simulink model "simscape_Example_20240513_1634"  (R2023b)
settings: Solver=ode23t  StartTime=0.0  StopTime=100  RelTol=1e-3
libraries: nesl_utility x10, fl_lib x8, ee_lib x4
settings Model: Creator=Patri  LastModifiedBy=Patri

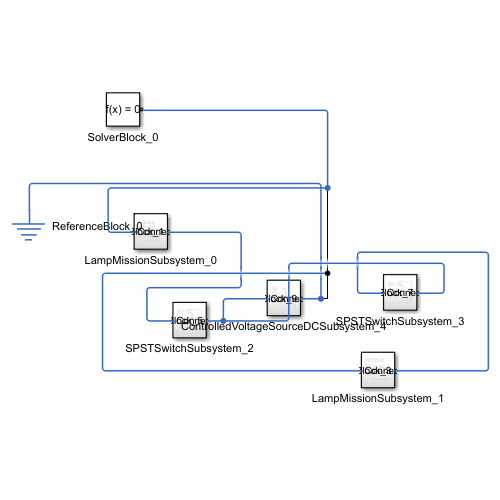
[thumbnail: Simulink's stored preview of the top-level diagram]
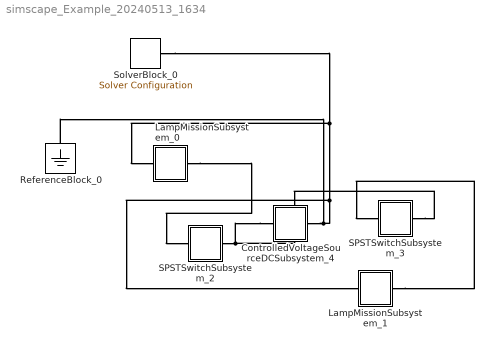
== system simscape_Example_20240513_1634 ==
  ControlledVoltageSourceDCSubsystem_4 : Subsystem
  LampMissionSubsystem_0 : Subsystem
  LampMissionSubsystem_1 : Subsystem
  ReferenceBlock_0 : fl_lib/Electrical/Electrical Elements/Electrical Reference
  SPSTSwitchSubsystem_2 : Subsystem
  SPSTSwitchSubsystem_3 : Subsystem
  SolverBlock_0 : nesl_utility/Solver Configuration  PhysicalDomain=network_engine_domain  SubClassName=solver  LeftPortType=input  RightPortType=generic  Tones=[]  Harmonics=[]  SimulateNoise=off  Profile=off  UseLocalSampling=off  EnableSwitchedLinearOptims=on  FrequencyDomain=off  UseCCode=off  RelTol=0.001  AbsTol=0.001  MinStep=1e-09  ToWorkspace=off  RevertToSquareIcSolve=off  NumHomotopyIterations=100  PhasorMode=off  PhasorModeNumHarmonics=1  ConsistencySolver=NEWTON_XTOL_AFTER_FTOL  IndexReductionMethod=DerivativeReplacement  DoDC=off  ResidualTolerance=1e-09  ConsistencyTolSource=GLOBAL  ConsistencyAbsTol=0.001  ConsistencyRelTol=0.001  ConsistencyTolFactor=0.001  UseLocalSolver=off  LocalSolverChoice=NE_BACKWARD_EULER_ADVANCER  ResolveIndetEquations=on  FunctionEvalNumThread=1  LocalSolverSampleTime=0.001  DoFixedCost=off  MaxNonlinIter=3  MaxModeIter=2  ComputeImpulses=off  ImpulseIterations=2  LinearAlgebra=auto  LinearAlgebraNumThread=0  EquationFormulation=NE_TIME_EF  DelaysMemoryBudget=1024  AutomaticFiltering=on  FilteringTimeConstant=0.001  PartitionStorageMethod=AS_NEEDED  PartitionMemoryBudget=1024  PartitionMethod=ROBUST  MultibodyUseLocalSolver=off  MultibodyLocalSolverChoice=ODE1  MultibodyLocalSolverSampleTime=0.001
  connections:
  ControlledVoltageSourceDCSubsystem_4/RConn1 -- SolverBlock_0/RConn1 -- LampMissionSubsystem_0/LConn1 -- LampMissionSubsystem_1/LConn1 -- ReferenceBlock_0/LConn1
  LampMissionSubsystem_0/RConn1 -- SPSTSwitchSubsystem_2/LConn1
  LampMissionSubsystem_1/RConn1 -- SPSTSwitchSubsystem_3/LConn1
  ControlledVoltageSourceDCSubsystem_4/LConn1 -- SPSTSwitchSubsystem_2/RConn1 -- SPSTSwitchSubsystem_3/RConn1

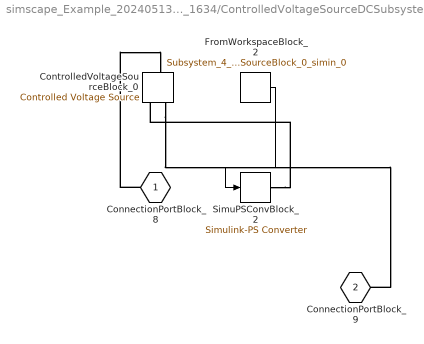
== system simscape_Example_20240513_1634/ControlledVoltageSourceDCSubsystem_4 ==
  ControlledVoltageSourceBlock_0 : fl_lib/Electrical/Electrical Sources/Controlled Voltage Source
  FromWorkspaceBlock_2 : FromWorkspace  VariableName=Subsystem_4_ControlledVoltageSourceBlock_0_simin_0
  SimuPSConvBlock_2 : nesl_utility/Simulink-PS Converter  PhysicalDomain=network_engine_domain  SubClassName=ps_input  LeftPortType=input  RightPortType=output  PseudoPeriodic=off  Frequencies=[]  NoiseDistribution=none  NoiseParameters=[]  Unit=1  AffineConversion=off  FilteringAndDerivatives=filter  SimscapeFilterOrder=1  InputFilterTimeConstant=0.001  UdotUserProvided=0
  ConnectionPortBlock_8 : PMIOPort  Side=Left
  ConnectionPortBlock_9 : PMIOPort  Port=2  Side=Right
  wires:
  FromWorkspaceBlock_2/1 -> SimuPSConvBlock_2/1
  connections:
  SimuPSConvBlock_2/RConn1 -- ControlledVoltageSourceBlock_0/RConn1
  ConnectionPortBlock_8/RConn1 -- ControlledVoltageSourceBlock_0/LConn1
  ControlledVoltageSourceBlock_0/RConn2 -- ConnectionPortBlock_9/RConn1

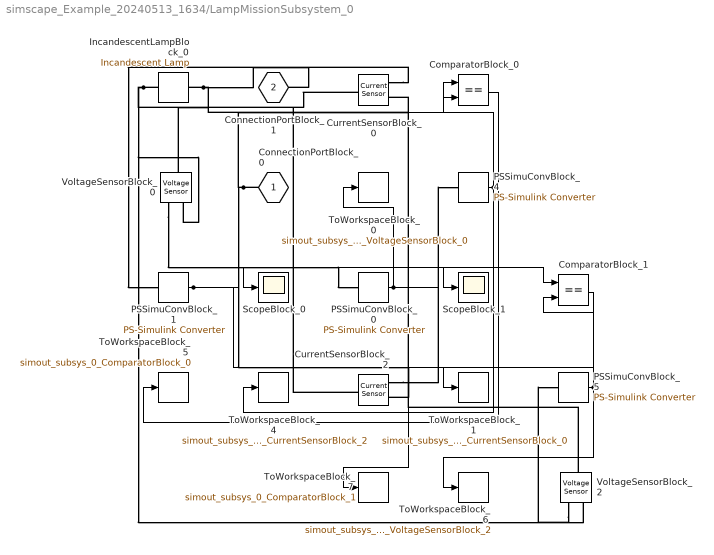
== system simscape_Example_20240513_1634/LampMissionSubsystem_0 ==
  ComparatorBlock_0 : RelationalOperator  Operator===  OutDataTypeStr=boolean  RndMeth=Simplest  InputSameDT=off
  ComparatorBlock_1 : RelationalOperator  Operator===  OutDataTypeStr=boolean  RndMeth=Simplest  InputSameDT=off
  CurrentSensorBlock_0 : fl_lib/Electrical/Electrical Sensors/Current Sensor
  CurrentSensorBlock_2 : fl_lib/Electrical/Electrical Sensors/Current Sensor
  IncandescentLampBlock_0 : ee_lib/Passive/Incandescent Lamp  R_param=ee.enum.passive.lampParam.specifyR  R0=0.15 Ohm  R1=1.0 Ohm  i0=70 A  i1=10 A  Vrated=12.0 V  alpha=0.004 1/K  tc=25 ms  initial_state=simscape.enum.onoff.off  enable_fault=simscape.enum.onoff.off  t_fault=inf s  R_fault=1e6 Ohm
      settings: InternalSimscapePortConfiguration="{\"Bottom\":[],\"Left\":[{\"id\":\"p\",\"label\":\"+\",\"type\":\"foundation.electrical.electrical\"}],\"Right\":[{\"id\":\"n\",\"label\":\"-\",\"type\":\"foundation.electrical.electrical\"}],\"Top\":[]}"
  PSSimuConvBlock_{0..1,4..5} (4 alike) : nesl_utility/PS-Simulink Converter  PhysicalDomain=network_engine_domain  SubClassName=ps_output  LeftPortType=input  RightPortType=output  PseudoPeriodic=off  Frequencies=[]  VectorFormat=inherit  Unit=inherit  AffineConversion=off
  ScopeBlock_0 : Scope
  ScopeBlock_1 : Scope
  ToWorkspaceBlock_0 : ToWorkspace  VariableName=simout_subsys_0_VoltageSensorBlock_0  SaveFormat=Structure With Time
  ToWorkspaceBlock_1 : ToWorkspace  VariableName=simout_subsys_0_CurrentSensorBlock_0  SaveFormat=Structure With Time
  ToWorkspaceBlock_4 : ToWorkspace  VariableName=simout_subsys_0_CurrentSensorBlock_2  SaveFormat=Structure With Time
  ToWorkspaceBlock_5 : ToWorkspace  VariableName=simout_subsys_0_ComparatorBlock_0  SaveFormat=Structure With Time  SampleTime=-1
  ToWorkspaceBlock_6 : ToWorkspace  VariableName=simout_subsys_0_VoltageSensorBlock_2  SaveFormat=Structure With Time
  ToWorkspaceBlock_7 : ToWorkspace  VariableName=simout_subsys_0_ComparatorBlock_1  SaveFormat=Structure With Time  SampleTime=-1
  VoltageSensorBlock_0 : fl_lib/Electrical/Electrical Sensors/Voltage Sensor
  VoltageSensorBlock_2 : fl_lib/Electrical/Electrical Sensors/Voltage Sensor
  ConnectionPortBlock_0 : PMIOPort  Side=Left
  ConnectionPortBlock_1 : PMIOPort  Port=2  Side=Right
  wires:
  PSSimuConvBlock_0/1 -> ToWorkspaceBlock_0/1, ScopeBlock_0/1, ComparatorBlock_1/1
  PSSimuConvBlock_1/1 -> ToWorkspaceBlock_1/1, ScopeBlock_1/1, ComparatorBlock_0/1
  PSSimuConvBlock_4/1 -> ToWorkspaceBlock_4/1, ComparatorBlock_0/2
  ComparatorBlock_0/1 -> ToWorkspaceBlock_5/1
  PSSimuConvBlock_5/1 -> ToWorkspaceBlock_6/1, ComparatorBlock_1/2
  ComparatorBlock_1/1 -> ToWorkspaceBlock_7/1
  connections:
  VoltageSensorBlock_0/RConn1 -- PSSimuConvBlock_0/LConn1
  VoltageSensorBlock_0/RConn2 -- IncandescentLampBlock_0/LConn1 -- CurrentSensorBlock_0/LConn1 -- CurrentSensorBlock_2/LConn1 -- VoltageSensorBlock_2/RConn2
  VoltageSensorBlock_0/LConn1 -- ConnectionPortBlock_1/RConn1 -- IncandescentLampBlock_0/RConn1 -- VoltageSensorBlock_2/LConn1
  CurrentSensorBlock_0/RConn1 -- PSSimuConvBlock_1/LConn1
  CurrentSensorBlock_0/RConn2 -- ConnectionPortBlock_0/RConn1 -- CurrentSensorBlock_2/RConn2
  CurrentSensorBlock_2/RConn1 -- PSSimuConvBlock_4/LConn1
  VoltageSensorBlock_2/RConn1 -- PSSimuConvBlock_5/LConn1

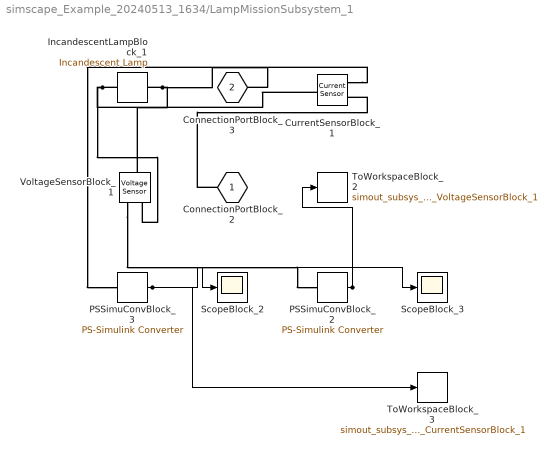
== system simscape_Example_20240513_1634/LampMissionSubsystem_1 ==
  CurrentSensorBlock_1 : fl_lib/Electrical/Electrical Sensors/Current Sensor
  IncandescentLampBlock_1 : ee_lib/Passive/Incandescent Lamp  R_param=ee.enum.passive.lampParam.specifyR  R0=0.15 Ohm  R1=1.0 Ohm  i0=70 A  i1=10 A  Vrated=12.0 V  alpha=0.004 1/K  tc=25 ms  initial_state=simscape.enum.onoff.off  enable_fault=simscape.enum.onoff.off  t_fault=inf s  R_fault=1e6 Ohm
      settings: InternalSimscapePortConfiguration="{\"Bottom\":[],\"Left\":[{\"id\":\"p\",\"label\":\"+\",\"type\":\"foundation.electrical.electrical\"}],\"Right\":[{\"id\":\"n\",\"label\":\"-\",\"type\":\"foundation.electrical.electrical\"}],\"Top\":[]}"
  PSSimuConvBlock_2 : nesl_utility/PS-Simulink Converter  PhysicalDomain=network_engine_domain  SubClassName=ps_output  LeftPortType=input  RightPortType=output  PseudoPeriodic=off  Frequencies=[]  VectorFormat=inherit  Unit=inherit  AffineConversion=off
  PSSimuConvBlock_3 : nesl_utility/PS-Simulink Converter  PhysicalDomain=network_engine_domain  SubClassName=ps_output  LeftPortType=input  RightPortType=output  PseudoPeriodic=off  Frequencies=[]  VectorFormat=inherit  Unit=inherit  AffineConversion=off
  ScopeBlock_2 : Scope
  ScopeBlock_3 : Scope
  ToWorkspaceBlock_2 : ToWorkspace  VariableName=simout_subsys_1_VoltageSensorBlock_1  SaveFormat=Structure With Time
  ToWorkspaceBlock_3 : ToWorkspace  VariableName=simout_subsys_1_CurrentSensorBlock_1  SaveFormat=Structure With Time
  VoltageSensorBlock_1 : fl_lib/Electrical/Electrical Sensors/Voltage Sensor
  ConnectionPortBlock_2 : PMIOPort  Side=Left
  ConnectionPortBlock_3 : PMIOPort  Port=2  Side=Right
  wires:
  PSSimuConvBlock_2/1 -> ToWorkspaceBlock_2/1, ScopeBlock_2/1
  PSSimuConvBlock_3/1 -> ToWorkspaceBlock_3/1, ScopeBlock_3/1
  connections:
  VoltageSensorBlock_1/RConn1 -- PSSimuConvBlock_2/LConn1
  VoltageSensorBlock_1/RConn2 -- IncandescentLampBlock_1/LConn1 -- CurrentSensorBlock_1/LConn1
  IncandescentLampBlock_1/RConn1 -- VoltageSensorBlock_1/LConn1 -- ConnectionPortBlock_3/RConn1
  CurrentSensorBlock_1/RConn1 -- PSSimuConvBlock_3/LConn1
  ConnectionPortBlock_2/RConn1 -- CurrentSensorBlock_1/RConn2

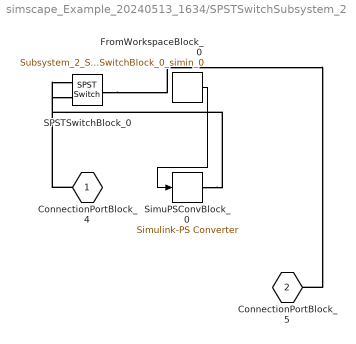
== system simscape_Example_20240513_1634/SPSTSwitchSubsystem_2 ==
  FromWorkspaceBlock_0 : FromWorkspace  VariableName=Subsystem_2_SPSTSwitchBlock_0_simin_0
  SPSTSwitchBlock_0 : ee_lib/Switches & Breakers/SPST Switch  R_closed=0.01 Ohm  G_open=1e-6 S  Threshold=0.5 V  Width=0 V  model_dynamics=0  t_on=1e-3 s  t_off=1e-3 s  initial_vT=0 V
      settings: InternalSimscapePortConfiguration="{\"Bottom\":[],\"Left\":[{\"id\":\"vT\",\"label\":\"vT\",\"type\":\"input\"},{\"id\":\"p\",\"label\":\"\",\"type\":\"foundation.electrical.electrical\"}],\"Right\":[{\"id\":\"n\",\"label\":\"\",\"type\":\"foundation.electrical.electrical\"}],\"Top\":[]}"
  SimuPSConvBlock_0 : nesl_utility/Simulink-PS Converter  PhysicalDomain=network_engine_domain  SubClassName=ps_input  LeftPortType=input  RightPortType=output  PseudoPeriodic=off  Frequencies=[]  NoiseDistribution=none  NoiseParameters=[]  Unit=1  AffineConversion=off  FilteringAndDerivatives=filter  SimscapeFilterOrder=1  InputFilterTimeConstant=0.001  UdotUserProvided=0
  ConnectionPortBlock_4 : PMIOPort  Side=Left
  ConnectionPortBlock_5 : PMIOPort  Port=2  Side=Right
  wires:
  FromWorkspaceBlock_0/1 -> SimuPSConvBlock_0/1
  connections:
  SimuPSConvBlock_0/RConn1 -- SPSTSwitchBlock_0/LConn1
  ConnectionPortBlock_4/RConn1 -- SPSTSwitchBlock_0/LConn2
  SPSTSwitchBlock_0/RConn1 -- ConnectionPortBlock_5/RConn1

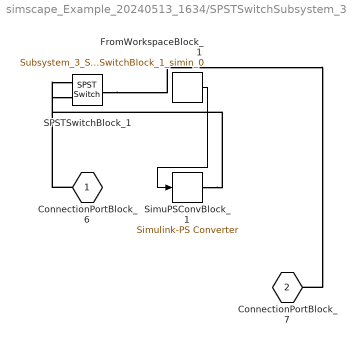
== system simscape_Example_20240513_1634/SPSTSwitchSubsystem_3 ==
  FromWorkspaceBlock_1 : FromWorkspace  VariableName=Subsystem_3_SPSTSwitchBlock_1_simin_0
  SPSTSwitchBlock_1 : ee_lib/Switches & Breakers/SPST Switch  R_closed=0.01 Ohm  G_open=1e-6 S  Threshold=0.5 V  Width=0 V  model_dynamics=0  t_on=1e-3 s  t_off=1e-3 s  initial_vT=0 V
      settings: InternalSimscapePortConfiguration="{\"Bottom\":[],\"Left\":[{\"id\":\"vT\",\"label\":\"vT\",\"type\":\"input\"},{\"id\":\"p\",\"label\":\"\",\"type\":\"foundation.electrical.electrical\"}],\"Right\":[{\"id\":\"n\",\"label\":\"\",\"type\":\"foundation.electrical.electrical\"}],\"Top\":[]}"
  SimuPSConvBlock_1 : nesl_utility/Simulink-PS Converter  PhysicalDomain=network_engine_domain  SubClassName=ps_input  LeftPortType=input  RightPortType=output  PseudoPeriodic=off  Frequencies=[]  NoiseDistribution=none  NoiseParameters=[]  Unit=1  AffineConversion=off  FilteringAndDerivatives=filter  SimscapeFilterOrder=1  InputFilterTimeConstant=0.001  UdotUserProvided=0
  ConnectionPortBlock_6 : PMIOPort  Side=Left
  ConnectionPortBlock_7 : PMIOPort  Port=2  Side=Right
  wires:
  FromWorkspaceBlock_1/1 -> SimuPSConvBlock_1/1
  connections:
  SimuPSConvBlock_1/RConn1 -- SPSTSwitchBlock_1/LConn1
  ConnectionPortBlock_6/RConn1 -- SPSTSwitchBlock_1/LConn2
  SPSTSwitchBlock_1/RConn1 -- ConnectionPortBlock_7/RConn1
